simulink model "sl_opspace_22a"  (R2022a)
settings: Solver=VariableStepAuto  StartTime=0.0  StopTime=2  RelTol=1e-3  EnableMultiTasking=on
PreLoadFcn:
  | if ~exist("puma", "var")
  |    [puma, conf] = loadrvcrobot("puma");
  | end
InitFcn:
  | fprintf("Parameters initialized in InitFcn\n");
  | 
  | if ~exist("puma", "var")
  |    [puma, conf] = loadrvcrobot("puma");
  | end
  | 
  | q = [0 pi/4 pi 0 -pi/4 0];
  | TE = se3(puma.getTransform(q, "link6"));
  | Sf = TE.rotm
  | 
  | % edit next 2 lines to change compliant motion axes
  | %  1 = freespace controlled motion
  | %  0 = constrained compliant motion
  | 
  | sigma_f = diag([1 1 0]);  % translation
  | sigma_t = diag([1 1 1]);  % rotation
  | 
  | omega = blkdiag( Sf'*sigma_t*Sf, Sf'*sigma_f*Sf)
  | omega_tilde = blkdiag( Sf'*(eye(3,3)-sigma_t)*Sf, Sf'*(eye(3,3)-sigma_f)*Sf)
undefined symbols (not defined in the file or in its folder): conf, massMatrixTask, puma, tformry, trvec2tform
libraries: robotmaniplib x4, robotcorelib x1, roblocks x1
Description:
  | Operational-space control system for a PUMA 560 robot.
  | 
  | Robotics, Vision and Control - 3rd Edition; Section 9.6.1
settings Model: Creator=corkep  LastModifiedBy=corkep
settings SolverCC: AlgebraicLoopSolver=TrustRegion  MaxZcPerStep=1
settings DataIOCC: LimitDataPoints=on  SaveFormat=Array  TimeSaveName=t  OutputSaveName=y  ReturnWorkspaceOutputsName=opspace
settings OptimizationCC: LifeSpan=inf
settings DebuggingCC: UnconnectedInputMsg=warning  UnconnectedOutputMsg=warning  UnconnectedLineMsg=warning  AllowSymbolicDim=off  SFUnexpectedBacktrackingDiag=warning  SFNoUnconditionalDefaultTransitionDiag=warning  SFExecutionAtInitializationDiag=none  SFMachineParentedDataDiag=warning  ArithmeticOperatorsInVariantConditions=warning
settings ModelReferenceCC: PropagateSignalLabelsOutOfModel=off
settings SFSimCC: SimUseLocalCustomCode=off  CustomCodeUndefinedFunction=UseInterfaceOnly
settings RTWCC: RTWUseLocalCustomCode=off
settings CodeAppCC: StateflowObjectComments=on
settings GRTTargetCC: TargetLangStandard=C89/C90 (ANSI)
settings ConfigComp: CovMetricSettings=dw  CovSaveCumulativeToWorkspaceVar=on  CovSaveSingleToWorkspaceVar=on  CovExternalEMLEnable=off

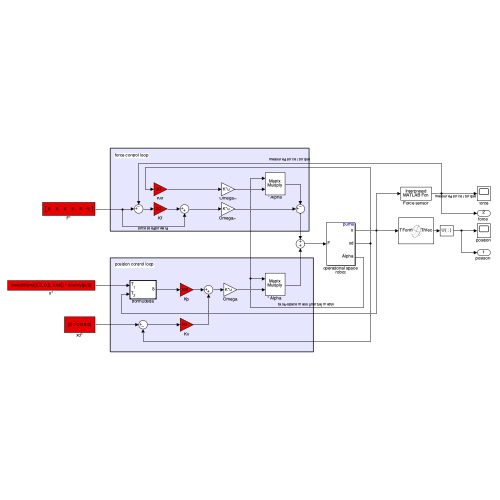
[thumbnail: Simulink's stored preview of the top-level diagram]
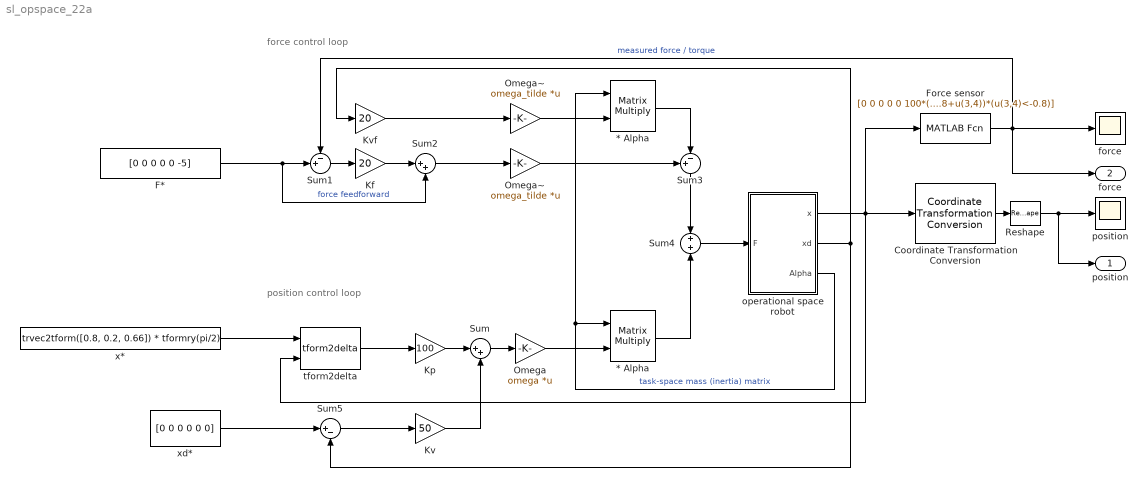
== system sl_opspace_22a ==
  note: position control loop
  note: force control loop
  * Alpha : Product  Multiplication=Matrix(*)
  "* Alpha " : Product  Multiplication=Matrix(*)
  Coordinate Transformation Conversion : robotcorelib/Coordinate Transformation Conversion  InputRepresentation=Homogeneous Transformation  InputEulerSequence=ZYX  ShowTrVecInputPort=on  OutputRepresentation=Translation Vector  OutputEulerSequence=ZYX  ShowTrVecOutputPort=on  SimulateUsing=Interpreted execution
  F* : Constant  Value=[0 0 0 0 0 -5]
  Force sensor : MATLABFcn  MATLABFcn=[0 0 0 0 0 100*(0.8+u(3,4))*(u(3,4)<-0.8)]
  Kf : Gain  Gain=20
  Kp : Gain  Gain=100
  Kv : Gain  Gain=50
  Kvf : Gain  Gain=20
  Omega : Gain  Gain=omega  Multiplication=Matrix(K*u)
  Omega~ : Gain  Gain=omega_tilde  Multiplication=Matrix(K*u)
  "Omega~ " : Gain  Gain=omega_tilde  Multiplication=Matrix(K*u)
  Reshape : Reshape
  Sum : Sum  Inputs=|++
  Sum1 : Sum  Inputs=-+|
  Sum2 : Sum  Inputs=|++
  Sum3 : Sum  Inputs=+-|
  Sum4 : Sum  Inputs=+|+
  Sum5 : Sum  Inputs=|+-
  force : Scope
  operational space robot : Subsystem  mask{robot=puma, q0=conf.qn}
      mask prompts: q0 "Initial joint angles"
      mask init:
      | sysName = get_param(gcb, 'robot')
      mask Display:
      | color('blue');
      | text(0.99, 0.99, sysName, 'horizontalAlignment', 'right', 'verticalAlignment','top');
      | 
      | color('black')
      | port_label('input', 1, 'F');
      | port_label('output', 1, 'x');
      | port_label('output', 2, 'xd');
      | port_label('output', 3, 'Alpha');
  position : Scope
  tform2delta : roblocks/tform2delta  SystemSampleTime=-1  VariantActivationTime=update diagram  Latency=0  AutoFrameSizeCalculation=off
  x* : Constant  Value=trvec2tform([0.8, 0.2, 0.66]) * tformry(pi/2)
  xd* : Constant  Value=[0 0 0 0 0 0]
  "position " : Outport
  "force " : Outport  Port=2
  wires:
  x*/1 -> tform2delta/1
  operational space robot/1(x) -> Coordinate Transformation Conversion/1, tform2delta/2, Force sensor/1
  operational space robot/3(Alpha) -> * Alpha/1, "* Alpha "/1  "task-space mass (inertia) matrix"
  Sum/1 -> Omega/1
  Kp/1 -> Sum/1
  tform2delta/1 -> Kp/1
  Kv/1 -> Sum/2
  operational space robot/2(xd) -> Kvf/1, Sum5/2
  Force sensor/1 -> "force "/1, force/1, Sum1/1  "measured force / torque"
  F*/1 -> Sum2/2, Sum1/2  "force feedforward"
  Sum1/1 -> Kf/1
  Kf/1 -> Sum2/1
  Kvf/1 -> Omega~/1
  Sum2/1 -> "Omega~ "/1
  Omega~/1 -> * Alpha/2
  * Alpha/1 -> Sum3/2
  "Omega~ "/1 -> Sum3/1
  "* Alpha "/1 -> Sum4/2
  Omega/1 -> "* Alpha "/2
  xd*/1 -> Sum5/1
  Sum5/1 -> Kv/1
  Sum4/1 -> operational space robot/1(F)
  Coordinate Transformation Conversion/1 -> Reshape/1
  Reshape/1 -> "position "/1, position/1
  Sum3/1 -> Sum4/1

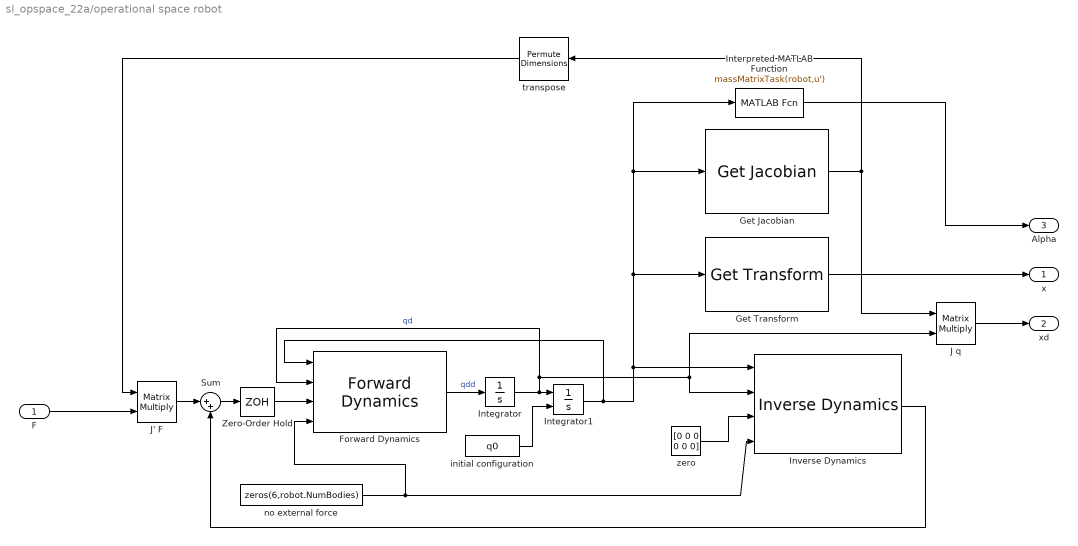
== system sl_opspace_22a/operational space robot ==
  F : Inport
  Forward Dynamics : robotmaniplib/Forward Dynamics  RigidBodyTree=robot  SimulateUsing=Interpreted execution
  Get Jacobian : robotmaniplib/Get Jacobian  RigidBodyTree=robot  EndEffector=link6  SimulateUsing=Interpreted execution
  Get Transform : robotmaniplib/Get Transform  RigidBodyTree=robot  SourceBody=link6  TargetBody=base  SimulateUsing=Interpreted execution
  Integrator : Integrator
  Integrator1 : Integrator  InitialConditionSource=external
  Interpreted MATLAB Function : MATLABFcn  MATLABFcn=massMatrixTask(robot,u')  OutputDimensions=[6 6]  Output1D=off
  Inverse Dynamics : robotmaniplib/Inverse Dynamics  RigidBodyTree=robot  SimulateUsing=Interpreted execution
  J q : Product  Multiplication=Matrix(*)
  J' F : Product  Multiplication=Matrix(*)
  Sum : Sum  Inputs=|++
  Zero-Order Hold : ZeroOrderHold  SampleTime=5e-3
  initial configuration : Constant  Value=q0
  no external force : Constant  Value=zeros(6,robot.NumBodies)
  transpose : PermuteDimensions
  zero : Constant  Value=[0 0 0 0 0 0]
  x : Outport
  xd : Outport  Port=2
  Alpha : Outport  Port=3
  wires:
  Interpreted MATLAB Function/1 -> Alpha/1
  Zero-Order Hold/1 -> Forward Dynamics/3
  Sum/1 -> Zero-Order Hold/1
  F/1 -> J' F/2
  transpose/1 -> J' F/1
  J' F/1 -> Sum/1
  zero/1 -> Inverse Dynamics/3
  Integrator1/1 -> Forward Dynamics/1, Inverse Dynamics/1, Get Transform/1, Get Jacobian/1, Interpreted MATLAB Function/1
  J q/1 -> xd/1
  Get Jacobian/1 -> J q/1, transpose/1
  Get Transform/1 -> x/1
  Inverse Dynamics/1 -> Sum/2
  initial configuration/1 -> Integrator1/2
  Forward Dynamics/1 -> Integrator/1  "qdd"
  Integrator/1 -> Inverse Dynamics/2, J q/2, Forward Dynamics/2, Integrator1/1  "qd"
  no external force/1 -> Forward Dynamics/4, Inverse Dynamics/4
